simulink model "roachf_2048ch"  (Simulink 7.5)
settings: Solver=ode45  StartTime=0.0  StopTime=10.0  RelTol=1e-3
undefined symbols (not defined in the file or in its folder): Down, quant, ROACH, Up
libraries: xbsIndex_r4 x1405, xps_library x39, xbsReplacements_r4 x14, casper_library_misc x13, casper_library_delays x4, casper_library_sources x4, simulink x1
(part 1 of 14)
settings Model: Creator=zaki  LastModifiedBy=zaki
settings DebuggingCC: StrictBusMsg=Warning

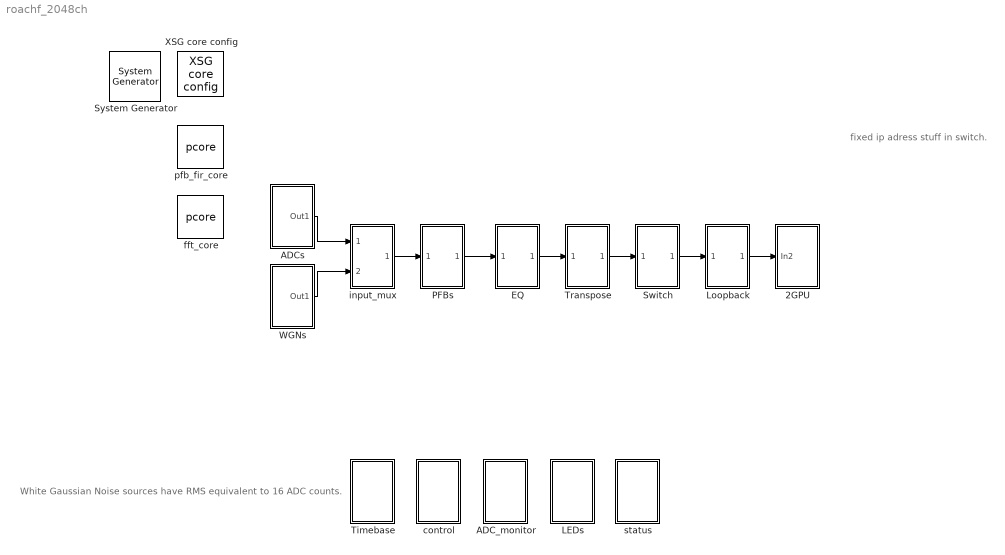
== system roachf_2048ch ==
  note: White Gaussian Noise
      | sources have RMS
      | equivalent to 16 ADC
      | counts.
  note: fixed ip adress stuff in switch.
  " System Generator" : xbsIndex_r4/ System Generator  Tag=genX  SystemSampleTime=-1  xilinxfamily=virtex5  part=xc5vsx95t  speed=-1  package=ff1136  synthesis_tool=XST  clock_wrapper=Clock Enables  directory=./roachf_2048ch/sysgen  proj_type=Project Navigator  Synth_file=XST Defaults  Impl_file=ISE Defaults  testbench=off  simulink_period=1  sysclk_period=5  dcm_input_clock_period=100  incr_netlist=off  trim_vbits=Everywhere in SubSystem  dbl_ovrd=According to Block Masks  core_generation=According to Block Masks  run_coregen=off  deprecated_control=off  eval_field=0  block_type=sysgen
      settings: block_version=10.1.3
  2GPU : Subsystem
  ADC_monitor : Subsystem
  ADCs : Subsystem
  EQ : Subsystem
  LEDs : Subsystem
  Loopback : Subsystem
  PFBs : Subsystem
  Switch : Subsystem
  Timebase : Subsystem
  Transpose : Subsystem
  WGNs : Subsystem
  XSG core config : xps_library/XSG core config  Tag=xps:xsg  SystemSampleTime=-1  hw_sys=ROACH:sx95t  ibob_linux=off  clk_src=adc0_clk  iBOB_clk_src=adc0_clk  BEE2_ctrl_clk_src=sys_clk  BEE2_usr_clk_src=sys_clk  ROACH_clk_src=adc0_clk  ROACH2_clk_src=adc0_clk  CORR_clk_src=sys_clk  gpio_clk_io_group=iBOB:sma  gpio_clk_bit_index=0  clk_rate=200  sample_period=1  synthesis_tool=XST  mpc_type=powerpc440_ext
  control : Subsystem
  fft_core : xps_library/pcore  Tag=xps:pcore  SystemSampleTime=-1  pcore_path=fft_core/fft_core.ngc
  input_mux : Subsystem
  pfb_fir_core : xps_library/pcore  Tag=xps:pcore  SystemSampleTime=-1  pcore_path=pfb_fir_core/pfb_fir_core.ngc
  status : Subsystem
  wires:
  ADCs/1(Out1) -> input_mux/1(In1)
  WGNs/1(Out1) -> input_mux/2(In2)
  input_mux/1(Out1) -> PFBs/1(In1)
  PFBs/1(Out1) -> EQ/1(In1)
  EQ/1(Out1) -> Transpose/1(In1)
  Transpose/1(Out1) -> Switch/1(In2)
  Switch/1(Out1) -> Loopback/1(In1)
  Loopback/1(Out1) -> 2GPU/1(In2)

== system roachf_2048ch/2GPU ==
  In2 : Inport
  10gbetxsnap : Subsystem  mask{nsamples=11}
      mask prompts: nsamples "Number of samples (2^?)"
  Constant1 : xbsIndex_r4/Constant  const=0  gui_display_data_type=Fixed-point  arith_type=Boolean  n_bits=16  bin_pt=14  preci_type=Single  exp_width=8  frac_width=24  explicit_period=on  period=1  equ=P=C  opselect=C  inp2=PCIN>>17  opr=+  inp1=P  carry=CIN  dbl_ovrd=off  block_type=constant
      settings: block_version=11.4
  Delay{,1..6} (7 alike) : xbsIndex_r4/Delay  rst=off  infoeditControl=Selection of Reset will increase slice count due to use of real FFs and instead of SRLs  en=off  latency=2  dbl_ovrd=off  reg_retiming=off  block_type=delay
  Inverter : xbsIndex_r4/Inverter  en=off  latency=0  dbl_ovrd=off  block_type=inv
      settings: block_version=11.4
  Inverter1 : xbsIndex_r4/Inverter  en=off  latency=0  dbl_ovrd=off  block_type=inv
  Logical : xbsIndex_r4/Logical  logical_function=AND  inputs=2  en=off  latency=0  precision=Full  arith_type=Unsigned  n_bits=16  bin_pt=0  align_bp=on  dbl_ovrd=off  block_type=logical
      settings: block_version=11.4
  Terminator : Terminator
  pack-it : Subsystem
  ten_GbE : xps_library/ten_GbE  Tag=xps:tengbe  SystemSampleTime=-1  port=ROACH:2  mac_lite=off  open_phy=off  show_param=off  pre_emph=3  swing=800  fab_en=off  fab_mac=0  fab_ip=0  fab_udp=0  fab_gate=0
  tag scope: gbe_gpu_led_rx=global, gbe_gpu_led_tx=global, gbe_gpu_led_up=global, gbe_gpu_rx_data=global, gbe_gpu_rx_eof=global, gbe_gpu_rx_ip=global, gbe_gpu_rx_port=global, gbe_gpu_rx_size=global, gbe_gpu_rx_valid=global, gbe_gpu_tx_ack=global
  wires:
  In2/1 -> Terminator/1
  [lb_mux_data] -> Delay/1
  [lb_mux_valid] -> Delay1/1
  [lb_mux_eof] -> Delay2/1
  [lb_mux_header] -> Delay3/1
  [lb_mux_flag] -> Delay4/1
  [lb_mux_err] -> Delay5/1
  [lb_mux_ip] -> Delay6/1
  [gpu_ip] -> ten_GbE/4
  [gpu_port] -> ten_GbE/5
  [data2gpu] -> ten_GbE/2
  pack-it/1(dataout) -> [data2gpu]
  pack-it/3(eof_out) -> [eof2gpu]
  pack-it/2(valid_out) -> [valid2gpu]
  [gbe_gpu_rst] -> ten_GbE/1
  Constant1/1 -> ten_GbE/8, ten_GbE/7
  [eof2gpu] -> ten_GbE/6
  ten_GbE/1 -> [gbe_gpu_led_up]
  ten_GbE/2 -> [gbe_gpu_led_rx]
  [gbe_gpu_disable] -> Inverter/1
  Inverter/1 -> Logical/1
  [valid2gpu] -> Logical/2
  Logical/1 -> 10gbetxsnap/2(valid_in), ten_GbE/3
  [data2gpu] -> 10gbetxsnap/1(data_in)
  [gpu_ip] -> 10gbetxsnap/3(ip_in)
  [eof2gpu] -> 10gbetxsnap/4(eof_in)
  [gbe_gpu_led_up] -> 10gbetxsnap/5(link_up)
  [gbe_gpu_led_tx] -> 10gbetxsnap/6(led_tx)
  [gbe_gpu_tx_ack] -> 10gbetxsnap/7(tx_ack)
  [gbe_gpu_tx_ack] -> Inverter1/1
  Delay/1 -> pack-it/1(data)
  Delay1/1 -> pack-it/2(valid)
  Delay2/1 -> pack-it/3(eof)
  Delay3/1 -> pack-it/4(header)
  Delay4/1 -> pack-it/5(flag)
  Delay5/1 -> pack-it/6(err)
  Delay6/1 -> pack-it/7(ip)
  ten_GbE/3 -> [gbe_gpu_led_tx]
  ten_GbE/4 -> [gbe_gpu_tx_ack]
  ten_GbE/5 -> [gbe_gpu_rx_data]
  ten_GbE/6 -> [gbe_gpu_rx_valid]
  ten_GbE/10 -> [gbe_gpu_rx_size]
  ten_GbE/7 -> [gbe_gpu_rx_ip]
  ten_GbE/8 -> [gbe_gpu_rx_port]
  ten_GbE/9 -> [gbe_gpu_rx_eof]
  Inverter1/1 -> 10gbetxsnap/8(tx_notack)

== system roachf_2048ch/ADC_monitor ==
  note: To provide a means for measuring the magnitude of the signals
      | coming in to each ADC channel, we have a "calc_adc_sum_sq"
      | block which uses a single multiplier, two accumulators, and two
      | regsiters to calculate the sum of 64K ADC samples and the sum
      | of squares of 64K ADC samples.  These can be used to calculate
      | the mean (aka DC offset) and standard deviation (aka RMS) of
      | the ADC inputs.
  note: adcN_levels are UFix_56_0.
      | The upper 16 bits are Fix_24_7 sum of samples.
      | The lower 32 bits are UFix_32_14 sum of squares.
  Counter : xbsIndex_r4/Counter  cnt_type=Free Running  cnt_to=Inf  operation=Up  start_count=0  cnt_by_val=1  arith_type=Unsigned  n_bits=16  bin_pt=0  load_pin=off  rst=off  en=off  explicit_period=off  period=1  dbl_ovrd=off  use_behavioral_HDL=off  implementation=Fabric  use_rpm=on  block_type=counter
      settings: xl_area=[0, 0, 0, 0, 0, 0, 0]
  Logical1 : xbsIndex_r4/Logical  logical_function=OR  inputs=8  en=off  latency=1  precision=Full  arith_type=Unsigned  n_bits=8  bin_pt=2  align_bp=on  dbl_ovrd=off  block_type=logical
      settings: xl_area=[0, 0, 0, 0, 0, 0, 0]
  Reinterpret{,1..7} (8 alike) : xbsIndex_r4/Reinterpret  force_arith_type=on  arith_type=Unsigned  force_bin_pt=on  bin_pt=0  block_type=reinterpret
      settings: infoedit="Changes signal type without altering the binary representation.   You can changed the signal between signed and unsigned, and relocate the binary point.<P><P>Hardware notes: In hardware this block costs nothing.<P><P>Example:  Suppose the input is 6 bits wide, signed, with 2 fractional bits, and the output is forced to unsigned with 0 fractional bits.  Then an input of -2.0 (1110.00 in binary 2's complement) becomes an output of 56 (111000 in binary)."  block_version=10.1.3
  Slice16 : xbsIndex_r4/Slice  nbits=1  boolean_output=on  mode=Upper Bit Location + Width  bit1=0  base1=MSB of Input  bit0=19  base0=LSB of Input  dbl_ovrd=off  block_type=slice
      settings: infoedit="Extracts a given range of bits from each input sample and presents it at the output.  The output type is ordinarily unsigned with binary point at zero, but can be Boolean when the slice is one bit wide.<P><P>Hardware notes: In hardware this block costs nothing."  block_version=10.1.3
  adc_clip_detect0 : Subsystem  mask{n_bits=8}
      mask prompts: n_bits "Number of ADC bits"
  adc_clip_detect1 : Subsystem  mask{n_bits=8}
      mask prompts: n_bits "Number of ADC bits"
  adc_clip_detect2 : Subsystem  mask{n_bits=8}
      mask prompts: n_bits "Number of ADC bits"
  adc_clip_detect3 : Subsystem  mask{n_bits=8}
      mask prompts: n_bits "Number of ADC bits"
  adc_clip_detect4 : Subsystem  mask{n_bits=8}
      mask prompts: n_bits "Number of ADC bits"
  adc_clip_detect5 : Subsystem  mask{n_bits=8}
      mask prompts: n_bits "Number of ADC bits"
  adc_clip_detect6 : Subsystem  mask{n_bits=8}
      mask prompts: n_bits "Number of ADC bits"
  adc_clip_detect7 : Subsystem  mask{n_bits=8}
      mask prompts: n_bits "Number of ADC bits"
  calc_adc_sum_sq0 : Subsystem
  calc_adc_sum_sq1 : Subsystem
  calc_adc_sum_sq2 : Subsystem
  calc_adc_sum_sq3 : Subsystem
  calc_adc_sum_sq4 : Subsystem
  calc_adc_sum_sq5 : Subsystem
  calc_adc_sum_sq6 : Subsystem
  calc_adc_sum_sq7 : Subsystem
  edge_detect : casper_library_misc/edge_detect  SystemSampleTime=-1  edge=Rising  polarity=Active High  x_in=[0 0.08 0.08 0.16 0.16 0.24 0.24 0.32 0.32 0.4]  y_in="[-1 -1  1  1  1  1  1  1  1  1]"  x_out=[0.6 0.68 0.68 0.76 0.76 0.84 0.84 0.92 0.92 1]  y_out="[-1 -1  1  1 -1 -1 -1 -1 -1 -1]"
  tag scope: adc_clip=global, in0_levels=global, in1_levels=global, in2_levels=global, in3_levels=global, in4_levels=global, in5_levels=global, in6_levels=global, in7_levels=global
  wires:
  [in0] -> calc_adc_sum_sq0/1(pol_in)
  calc_adc_sum_sq1/1(sum_sumsq) -> Reinterpret1/1
  calc_adc_sum_sq2/1(sum_sumsq) -> Reinterpret2/1
  calc_adc_sum_sq3/1(sum_sumsq) -> Reinterpret3/1
  edge_detect/1 -> calc_adc_sum_sq0/2(accum_rst), calc_adc_sum_sq1/2(accum_rst), calc_adc_sum_sq2/2(accum_rst), calc_adc_sum_sq3/2(accum_rst), calc_adc_sum_sq4/2(accum_rst), calc_adc_sum_sq5/2(accum_rst), calc_adc_sum_sq6/2(accum_rst), calc_adc_sum_sq7/2(accum_rst)
  [in1] -> calc_adc_sum_sq1/1(pol_in)
  [in2] -> calc_adc_sum_sq2/1(pol_in)
  [in3] -> calc_adc_sum_sq3/1(pol_in)
  Counter/1 -> Slice16/1
  Slice16/1 -> edge_detect/1
  calc_adc_sum_sq4/1(sum_sumsq) -> Reinterpret4/1
  [in4] -> calc_adc_sum_sq4/1(pol_in)
  calc_adc_sum_sq5/1(sum_sumsq) -> Reinterpret5/1
  calc_adc_sum_sq6/1(sum_sumsq) -> Reinterpret6/1
  calc_adc_sum_sq7/1(sum_sumsq) -> Reinterpret7/1
  [in5] -> calc_adc_sum_sq5/1(pol_in)
  [in6] -> calc_adc_sum_sq6/1(pol_in)
  [in7] -> calc_adc_sum_sq7/1(pol_in)
  Reinterpret/1 -> [in0_levels]
  Reinterpret1/1 -> [in1_levels]
  Reinterpret2/1 -> [in2_levels]
  Reinterpret3/1 -> [in3_levels]
  Reinterpret4/1 -> [in4_levels]
  Reinterpret5/1 -> [in5_levels]
  Reinterpret6/1 -> [in6_levels]
  Reinterpret7/1 -> [in7_levels]
  calc_adc_sum_sq0/1(sum_sumsq) -> Reinterpret/1
  [adc0] -> adc_clip_detect0/1(adc_in)
  [adc1] -> adc_clip_detect1/1(adc_in)
  [adc2] -> adc_clip_detect2/1(adc_in)
  [adc3] -> adc_clip_detect3/1(adc_in)
  [adc4] -> adc_clip_detect4/1(adc_in)
  [adc5] -> adc_clip_detect5/1(adc_in)
  [adc6] -> adc_clip_detect6/1(adc_in)
  [adc7] -> adc_clip_detect7/1(adc_in)
  adc_clip_detect0/1(clip) -> Logical1/1
  adc_clip_detect1/1(clip) -> Logical1/2
  adc_clip_detect2/1(clip) -> Logical1/3
  adc_clip_detect3/1(clip) -> Logical1/4
  adc_clip_detect4/1(clip) -> Logical1/5
  adc_clip_detect5/1(clip) -> Logical1/6
  adc_clip_detect6/1(clip) -> Logical1/7
  adc_clip_detect7/1(clip) -> Logical1/8
  Logical1/1 -> [adc_clip]

== system roachf_2048ch/ADCs ==
  Band-Limited White Noise : simulink/Sources/Band-Limited White Noise  SystemSampleTime=-1  Cov=[0.1]  Ts=0.1  seed=[23341]
  Constant : Constant  Value=0
  Constant1 : Constant
  Constant2 : Constant  Value=0
  Mux : Mux  Inputs=2
  Pulse Generator : DiscretePulseGenerator  Amplitude=1  Period=2^27  PulseWidth=1  PhaseDelay=0  SampleTime=1
  Terminator11 : Terminator
  Terminator12 : Terminator
  quadc0 : xps_library/quadc  Tag=xps:quadc  SystemSampleTime=-1  adc_brd=0  adc_clk_rate=200
  quadc1 : xps_library/quadc  Tag=xps:quadc  SystemSampleTime=-1  adc_brd=1  adc_clk_rate=200
  Out1 : Outport
  tag scope: adc0=global, adc1=global, adc2=global, adc3=global, adc4=global, adc5=global, adc6=global, adc7=global, sync_adc0=global, sync_adc1=global
  wires:
  quadc0/1 -> [adc0]
  quadc0/2 -> [adc1]
  quadc0/3 -> [adc2]
  quadc0/4 -> [adc3]
  quadc0/6 -> [sync_adc0]
  quadc1/1 -> [adc4]
  quadc1/2 -> [adc5]
  quadc1/3 -> [adc6]
  quadc1/4 -> [adc7]
  quadc1/6 -> [sync_adc1]
  Band-Limited White Noise/1 -> quadc1/4, quadc1/3, quadc1/2, quadc1/1, quadc0/4, quadc0/3, quadc0/2, quadc0/1
  Pulse Generator/1 -> quadc0/6, quadc1/6
  Constant1/1 -> quadc0/5, quadc1/5
  quadc0/5 -> Terminator11/1
  quadc1/5 -> Terminator12/1
  Mux/1 -> Out1/1
  Constant/1 -> Mux/1
  Constant2/1 -> Mux/2

== system roachf_2048ch/EQ ==
  note: Next, we reduce the bitwidth out of the FFT to 4 bits to save resources.
      | This must be done very carefully to avoid losing too much information.
      | Firstly, this conversion is done using "Round to Even" and saturation
      | logic to avoid introducing DC offsets, wrapping, and other ugly quantizaton
      | effects.  Secondly, the "equalizer" allows each frequency channel of the
      | FFT to be scaled by a different number.  This allows passbands which are
      | not flat to be flattened digitally to allow for optimal quantization to 4 bits.
      | These coefficients can also be updated dynamically for gain control.
      | Coefficients can be dynamically written into the "equalizer" by
      | specifying the channel ("coeff_addr") and the value of the
      | coefficient ("coeff"), and then using "coeff_en" to write the
      | new coefficient into the equalization table.
  note: eq_mon will monitor eq0, which consists of
      | in0 spectrum followed by in1 spectrum
  In1 : Inport
  Concat3 : xbsIndex_r4/Concat  num_inputs=4  dbl_ovrd=off  block_type=concat
      settings: block_version=10.1.3
  Logical5 : xbsIndex_r4/Logical  logical_function=OR  inputs=4  en=off  latency=0  precision=Full  arith_type=Unsigned  n_bits=8  bin_pt=2  align_bp=on  dbl_ovrd=off  block_type=logical
      settings: xl_area=[0, 0, 0, 0, 0, 0, 0]
  Terminator13 : Terminator
  Terminator14 : Terminator
  Terminator15 : Terminator
  eq0 : Subsystem
  eq1 : Subsystem
  eq2 : Subsystem
  eq3 : Subsystem
  Out1 : Outport
  tag scope: eq0=global, eq1=global, eq2=global, eq3=global, eq_clip0=global, eq_clip1=global, eq_clip2=global, eq_clip3=global, eq_clip=global, eq_mon=global, eq_out=global, sync_rnd=global
  wires:
  eq0/1(dout) -> [eq0], [eq_mon]
  eq0/2(sync_out) -> [sync_rnd]
  [fft0] -> eq0/1(in)
  [eq_data_0] -> eq0/3(coeff)
  [eq_en_0] -> eq0/4(coeff_we)
  eq0/3(clip) -> [eq_clip0]
  Logical5/1 -> [eq_clip]
  Concat3/1 -> [eq_out]
  [eq_clip0] -> Logical5/1
  [eq_clip1] -> Logical5/2
  [sync_fft0] -> eq0/2(sync)
  [eq_addr_0] -> eq0/5(coeff_addr)
  [fft1] -> eq1/1(in)
  [sync_fft0] -> eq1/2(sync)
  [eq_data_1] -> eq1/3(coeff)
  [eq_en_1] -> eq1/4(coeff_we)
  [eq_addr_1] -> eq1/5(coeff_addr)
  [fft2] -> eq2/1(in)
  [sync_fft0] -> eq2/2(sync)
  [eq_data_2] -> eq2/3(coeff)
  [eq_en_2] -> eq2/4(coeff_we)
  [eq_addr_2] -> eq2/5(coeff_addr)
  [fft3] -> eq3/1(in)
  [sync_fft0] -> eq3/2(sync)
  [eq_data_3] -> eq3/3(coeff)
  [eq_en_3] -> eq3/4(coeff_we)
  [eq_addr_3] -> eq3/5(coeff_addr)
  eq1/1(dout) -> [eq1]
  eq1/2(sync_out) -> Terminator13/1
  eq1/3(clip) -> [eq_clip1]
  eq2/1(dout) -> [eq2]
  eq2/2(sync_out) -> Terminator14/1
  eq2/3(clip) -> [eq_clip2]
  eq3/1(dout) -> [eq3]
  eq3/2(sync_out) -> Terminator15/1
  eq3/3(clip) -> [eq_clip3]
  [eq_clip2] -> Logical5/3
  [eq_clip3] -> Logical5/4
  [eq0] -> Concat3/1
  [eq1] -> Concat3/2
  [eq2] -> Concat3/3
  [eq3] -> Concat3/4
  In1/1 -> Out1/1

== system roachf_2048ch/LEDs ==
  Terminator{1..3,27} (4 alike) : Terminator
  led1_arm : xps_library/gpio  Tag=xps:gpio  SystemSampleTime=-1  io_group=ROACH:led  io_dir=out  arith_type=Boolean  bitwidth=1  bin_pt=0  bit_index=0  sample_period=1  use_single_ended=off  use_ddr=off  reg_iob=on  reg_clk_phase=0  termination=None
      link override convert: arith_type=Boolean  n_bits=1  bin_pt=0
  led2_sync : xps_library/gpio  Tag=xps:gpio  SystemSampleTime=-1  io_group=ROACH:led  io_dir=out  arith_type=Boolean  bitwidth=1  bin_pt=0  bit_index=1  sample_period=1  use_single_ended=off  use_ddr=off  reg_iob=on  reg_clk_phase=0  termination=None
      link override convert: arith_type=Boolean  n_bits=1  bin_pt=0
  led4_eq_clip : xps_library/gpio  Tag=xps:gpio  SystemSampleTime=-1  io_group=ROACH:led  io_dir=out  arith_type=Boolean  bitwidth=1  bin_pt=0  bit_index=2  sample_period=1  use_single_ended=off  use_ddr=off  reg_iob=on  reg_clk_phase=0  termination=None
      link override convert: arith_type=Boolean  n_bits=1  bin_pt=0
  led5_adc_clip : xps_library/gpio  Tag=xps:gpio  SystemSampleTime=-1  io_group=ROACH:led  io_dir=out  arith_type=Boolean  bitwidth=1  bin_pt=0  bit_index=3  sample_period=1  use_single_ended=off  use_ddr=off  reg_iob=on  reg_clk_phase=0  termination=None
      link override convert: arith_type=Boolean  n_bits=1  bin_pt=0
  pulse_ext2 : Subsystem  mask{pulse_len=2^23}
      mask prompts: pulse_len "Length of Pulse"
      mask init:
      | bits = ceil(log2(pulse_len+1));
  pulse_ext3 : Subsystem  mask{pulse_len=2^18}
      mask prompts: pulse_len "Length of Pulse"
      mask init:
      | bits = ceil(log2(pulse_len+1));
  pulse_ext4 : Subsystem  mask{pulse_len=2^18}
      mask prompts: pulse_len "Length of Pulse"
      mask init:
      | bits = ceil(log2(pulse_len+1));
  wires:
  pulse_ext2/1(out) -> led2_sync/1
  [sync_gen] -> pulse_ext2/1(in)
  [armed] -> led1_arm/1
  pulse_ext4/1(out) -> led4_eq_clip/1
  [eq_clip] -> pulse_ext4/1(in)
  led1_arm/1 -> Terminator27/1
  led4_eq_clip/1 -> Terminator2/1
  led2_sync/1 -> Terminator3/1
  [adc_clip] -> pulse_ext3/1(in)
  pulse_ext3/1(out) -> led5_adc_clip/1
  led5_adc_clip/1 -> Terminator1/1

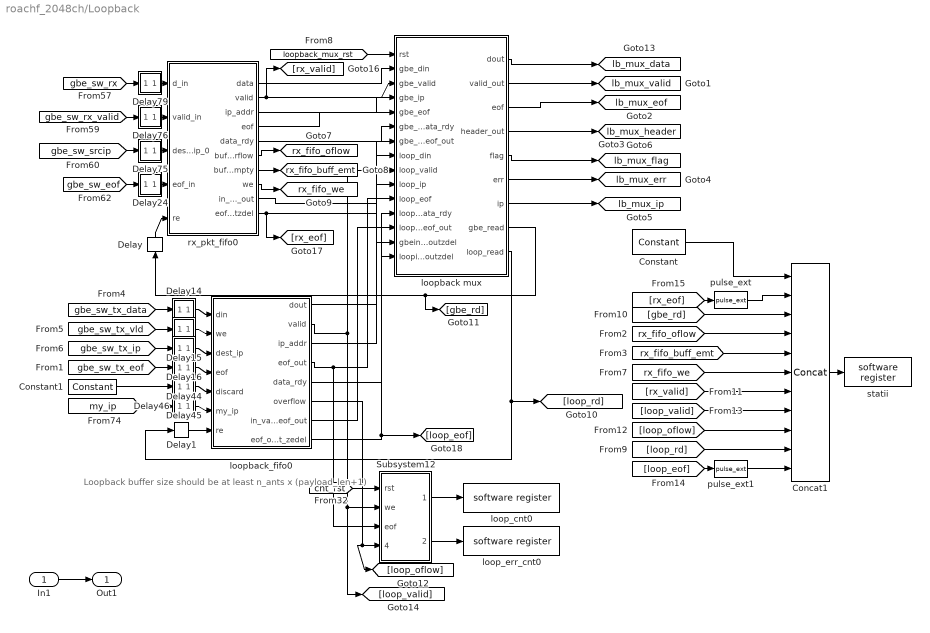
== system roachf_2048ch/Loopback ==
  note: Loopback buffer size should be at least
      | n_ants x (payload_len+1)
  In1 : Inport
  Concat1 : xbsIndex_r4/Concat  num_inputs=11  dbl_ovrd=off  block_type=concat
  Constant : xbsIndex_r4/Constant  const=0  gui_display_data_type=Fixed-point  arith_type=Unsigned  n_bits=22  bin_pt=0  preci_type=Single  exp_width=8  frac_width=24  explicit_period=on  period=1  equ=P=C  opselect=C  inp2=PCIN>>17  opr=+  inp1=P  carry=CIN  dbl_ovrd=off  block_type=constant
      settings: block_version=11.4
  Constant1 : xbsIndex_r4/Constant  const=0  gui_display_data_type=Boolean  arith_type=Boolean  n_bits=1  bin_pt=0  preci_type=Single  exp_width=8  frac_width=24  explicit_period=on  period=1  equ=P=C  opselect=C  inp2=PCIN>>17  opr=+  inp1=P  carry=CIN  dbl_ovrd=off  block_type=constant
      settings: block_version=11.4
  Delay : xbsIndex_r4/Delay  rst=off  infoeditControl=Selection of Reset will increase slice count due to use of real FFs and instead of SRLs  en=off  latency=1  dbl_ovrd=off  reg_retiming=off  block_type=delay
  Delay1 : xbsIndex_r4/Delay  rst=off  infoeditControl=Selection of Reset will increase slice count due to use of real FFs and instead of SRLs  en=off  latency=1  dbl_ovrd=off  reg_retiming=off  block_type=delay
  Delay14 : Subsystem  AncestorBlock=casper_library/Delays/pipeline  mask(pipeline){latency=1}
      mask help:
      | An explicitly laid-out delay line to avoid mapping to SRL16s
      | for use in pipelining to help achieve timing closure.
      mask init:
      | pipeline_init(gcb, 'latency', latency);
      mask Display:
      | port_label('input', 1, 'd');
      | port_label('output', 1, 'q');
      | disp(['Z^-', num2str(latency)]);
  Delay15 : Subsystem  AncestorBlock=casper_library/Delays/pipeline  mask(pipeline){latency=1}
      mask help:
      | An explicitly laid-out delay line to avoid mapping to SRL16s
      | for use in pipelining to help achieve timing closure.
      mask init:
      | pipeline_init(gcb, 'latency', latency);
      mask Display:
      | port_label('input', 1, 'd');
      | port_label('output', 1, 'q');
      | disp(['Z^-', num2str(latency)]);
  Delay16 : Subsystem  AncestorBlock=casper_library/Delays/pipeline  mask(pipeline){latency=1}
      mask help:
      | An explicitly laid-out delay line to avoid mapping to SRL16s
      | for use in pipelining to help achieve timing closure.
      mask init:
      | pipeline_init(gcb, 'latency', latency);
      mask Display:
      | port_label('input', 1, 'd');
      | port_label('output', 1, 'q');
      | disp(['Z^-', num2str(latency)]);
  Delay24 : Subsystem  AncestorBlock=casper_library/Delays/pipeline  mask(pipeline){latency=1}
      mask help:
      | An explicitly laid-out delay line to avoid mapping to SRL16s
      | for use in pipelining to help achieve timing closure.
      mask init:
      | pipeline_init(gcb, 'latency', latency);
      mask Display:
      | port_label('input', 1, 'd');
      | port_label('output', 1, 'q');
      | disp(['Z^-', num2str(latency)]);
  Delay44 : Subsystem  AncestorBlock=casper_library/Delays/pipeline  mask(pipeline){latency=1}
      mask help:
      | An explicitly laid-out delay line to avoid mapping to SRL16s
      | for use in pipelining to help achieve timing closure.
      mask init:
      | pipeline_init(gcb, 'latency', latency);
      mask Display:
      | port_label('input', 1, 'd');
      | port_label('output', 1, 'q');
      | disp(['Z^-', num2str(latency)]);
  Delay45 : Subsystem  AncestorBlock=casper_library/Delays/pipeline  mask(pipeline){latency=1}
      mask help:
      | An explicitly laid-out delay line to avoid mapping to SRL16s
      | for use in pipelining to help achieve timing closure.
      mask init:
      | pipeline_init(gcb, 'latency', latency);
      mask Display:
      | port_label('input', 1, 'd');
      | port_label('output', 1, 'q');
      | disp(['Z^-', num2str(latency)]);
  Delay46 : Subsystem  AncestorBlock=casper_library/Delays/pipeline  mask(pipeline){latency=1}
      mask help:
      | An explicitly laid-out delay line to avoid mapping to SRL16s
      | for use in pipelining to help achieve timing closure.
      mask init:
      | pipeline_init(gcb, 'latency', latency);
      mask Display:
      | port_label('input', 1, 'd');
      | port_label('output', 1, 'q');
      | disp(['Z^-', num2str(latency)]);
  Delay75 : Subsystem  AncestorBlock=casper_library/Delays/pipeline  mask(pipeline){latency=1}
      mask help:
      | An explicitly laid-out delay line to avoid mapping to SRL16s
      | for use in pipelining to help achieve timing closure.
      mask init:
      | pipeline_init(gcb, 'latency', latency);
      mask Display:
      | port_label('input', 1, 'd');
      | port_label('output', 1, 'q');
      | disp(['Z^-', num2str(latency)]);
  Delay76 : Subsystem  AncestorBlock=casper_library/Delays/pipeline  mask(pipeline){latency=1}
      mask help:
      | An explicitly laid-out delay line to avoid mapping to SRL16s
      | for use in pipelining to help achieve timing closure.
      mask init:
      | pipeline_init(gcb, 'latency', latency);
      mask Display:
      | port_label('input', 1, 'd');
      | port_label('output', 1, 'q');
      | disp(['Z^-', num2str(latency)]);
  Delay79 : Subsystem  AncestorBlock=casper_library/Delays/pipeline  mask(pipeline){latency=1}
      mask help:
      | An explicitly laid-out delay line to avoid mapping to SRL16s
      | for use in pipelining to help achieve timing closure.
      mask init:
      | pipeline_init(gcb, 'latency', latency);
      mask Display:
      | port_label('input', 1, 'd');
      | port_label('output', 1, 'q');
      | disp(['Z^-', num2str(latency)]);
  Subsystem12 : Subsystem
  loop_cnt0 : xps_library/software register  Tag=xps:sw_reg  SystemSampleTime=-1  io_dir=To Processor  arith_type=Unsigned  bitwidth=32  bin_pt=0  sample_period=1  gw_name=roachf_2048ch_Loopback_loop_cnt0_user_data_in
      link override convert: arith_type=Unsigned  n_bits=32  bin_pt=0
  loop_err_cnt0 : xps_library/software register  Tag=xps:sw_reg  SystemSampleTime=-1  io_dir=To Processor  arith_type=Unsigned  bitwidth=32  bin_pt=0  sample_period=1  gw_name=roachf_2048ch_Loopback_loop_err_cnt0_user_data_in
      link override convert: arith_type=Unsigned  n_bits=32  bin_pt=0
  loopback mux : Subsystem
  loopback_fifo0 : Subsystem
  pulse_ext : casper_library_misc/pulse_ext  SystemSampleTime=-1  pulse_len=512
  pulse_ext1 : casper_library_misc/pulse_ext  SystemSampleTime=-1  pulse_len=512
  rx_pkt_fifo0 : Subsystem
      settings: AttributesFormatString=|
      | Max 1024 data words.
      | Max 32 pkts.
  statii : xps_library/software register  Tag=xps:sw_reg  SystemSampleTime=-1  io_dir=To Processor  arith_type=Unsigned  bitwidth=32  bin_pt=0  sample_period=1  gw_name=roachf_2048ch_Loopback_statii_user_data_in
      link override convert: arith_type=Unsigned  n_bits=32  bin_pt=0
  Out1 : Outport
  tag scope: lb_mux_data=global, lb_mux_eof=global, lb_mux_err=global, lb_mux_flag=global, lb_mux_header=global, lb_mux_ip=global, lb_mux_valid=global, rx_fifo_buff_emt=global, rx_fifo_oflow=global, rx_fifo_we=global
  wires:
  loopback_fifo0/2(valid) -> loopback mux/9(loop_valid), Subsystem12/2(we), [loop_valid]
  rx_pkt_fifo0/1(data) -> loopback mux/2(gbe_din)
  rx_pkt_fifo0/2(valid) -> loopback mux/3(gbe_valid), [rx_valid]
  [cnt_rst] -> Subsystem12/1(rst)
  Subsystem12/2(err_cnt) -> loop_err_cnt0/1
  Subsystem12/1(rx_cnt) -> loop_cnt0/1
  [loopback_mux_rst] -> loopback mux/1(rst)
  [gbe_sw_srcip] -> Delay75/1(d)
  [gbe_sw_rx_valid] -> Delay76/1(d)
  [gbe_sw_rx] -> Delay79/1(d)
  [gbe_sw_eof] -> Delay24/1(d)
  Delay79/1(q) -> rx_pkt_fifo0/1(d_in)
  Delay76/1(q) -> rx_pkt_fifo0/2(valid_in)
  Delay75/1(q) -> rx_pkt_fifo0/3(dest_ip_0)
  Delay24/1(q) -> rx_pkt_fifo0/4(eof_in)
  [my_ip] -> Delay46/1(d)
  [gbe_sw_tx_data] -> Delay14/1(d)
  [gbe_sw_tx_vld] -> Delay15/1(d)
  [gbe_sw_tx_ip] -> Delay16/1(d)
  [gbe_sw_tx_eof] -> Delay44/1(d)
  Constant1/1 -> Delay45/1(d)
  Delay14/1(q) -> loopback_fifo0/1(din)
  Delay15/1(q) -> loopback_fifo0/2(we)
  Delay16/1(q) -> loopback_fifo0/3(dest_ip)
  Delay44/1(q) -> loopback_fifo0/4(eof)
  Delay45/1(q) -> loopback_fifo0/5(discard)
  Delay46/1(q) -> loopback_fifo0/6(my_ip)
  In1/1 -> Out1/1
  loopback mux/1(dout) -> [lb_mux_data]
  loopback mux/2(valid_out) -> [lb_mux_valid]
  loopback mux/5(flag) -> [lb_mux_flag]
  loopback mux/6(err) -> [lb_mux_err]
  Concat1/1 -> statii/1
  loopback mux/3(eof) -> [lb_mux_eof]
  loopback mux/4(header_out) -> [lb_mux_header]
  loopback mux/7(ip) -> [lb_mux_ip]
  loopback mux/9(loop_read) -> Delay1/1, [loop_rd]
  loopback_fifo0/4(eof_out) -> Subsystem12/3(eof), loopback mux/11(loop_eof)
  loopback_fifo0/6(overflow) -> Subsystem12/4(overflow), [loop_oflow]
  rx_pkt_fifo0/6(buffer_overflow) -> [rx_fifo_oflow]
  rx_pkt_fifo0/7(buffer_empty) -> [rx_fifo_buff_emt]
  rx_pkt_fifo0/8(we) -> [rx_fifo_we]
  loopback mux/8(gbe_read) -> Delay/1, [gbe_rd]
  rx_pkt_fifo0/4(eof) -> loopback mux/5(gbe_eof)
  rx_pkt_fifo0/3(ip_addr) -> loopback mux/4(gbe_ip)
  rx_pkt_fifo0/5(data_rdy) -> loopback mux/6(gbe_data_rdy)
  rx_pkt_fifo0/9(in_valid_eof_out) -> loopback mux/7(gbe_in_valid_eof_out)
  loopback_fifo0/1(dout) -> loopback mux/8(loop_din)
  loopback_fifo0/3(ip_addr) -> loopback mux/10(loop_ip)
  loopback_fifo0/5(data_rdy) -> loopback mux/12(loop_data_rdy)
  loopback_fifo0/7(in_valid_eof_out) -> loopback mux/13(loop_in_valid_eof_out)
  rx_pkt_fifo0/10(eofoutzdel) -> loopback mux/14(gbeineofoutzdel), [rx_eof]
  loopback_fifo0/8(eof_out_zedel) -> loopback mux/15(loopineofoutzdel), [loop_eof]
  Delay/1 -> rx_pkt_fifo0/5(re)
  Delay1/1 -> loopback_fifo0/7(re)
  [rx_eof] -> pulse_ext/1
  [loop_eof] -> pulse_ext1/1
  pulse_ext1/1 -> Concat1/11
  [loop_rd] -> Concat1/10
  [loop_oflow] -> Concat1/9
  [loop_valid] -> Concat1/8
  [rx_valid] -> Concat1/7
  [rx_fifo_we] -> Concat1/6
  [rx_fifo_buff_emt] -> Concat1/5
  [rx_fifo_oflow] -> Concat1/4
  [gbe_rd] -> Concat1/3
  pulse_ext/1 -> Concat1/2
  Constant/1 -> Concat1/1

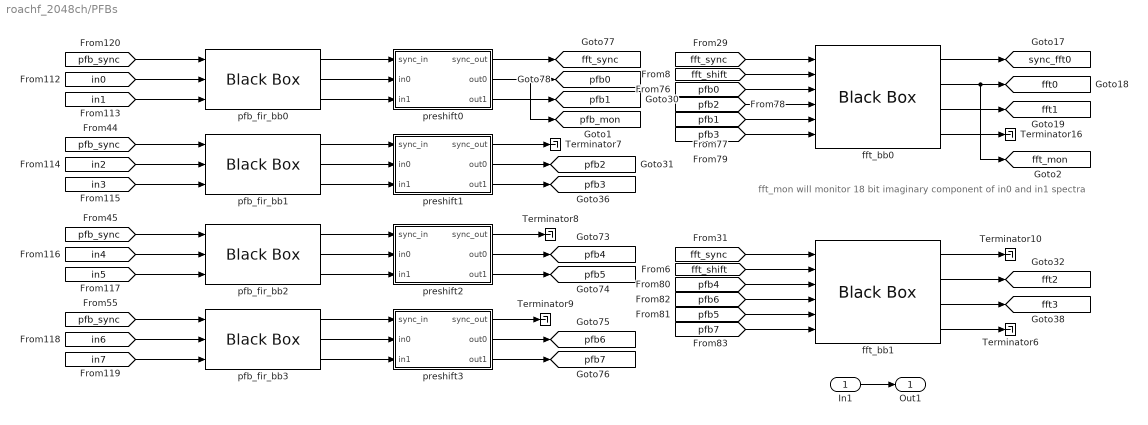
== system roachf_2048ch/PFBs ==
  note: fft_mon will monitor 18 bit imaginary component of in0 and in1 spectra
  In1 : Inport
  Terminator{6..10,16} (6 alike) : Terminator
  fft_bb0 : xbsIndex_r4/Black Box  init_code=fft_core_config  sim_method=Inactive  verbose=off  block_type=blackbox2
      settings: infoedit="Incorporates black box HDL and simulation model into a System Generator design.<P><P>You must supply a Black Box with certain information about the HDL component you would like to bring into System Generator. This information is provided through a Matlab function.<P><P>When \"Simulation mode\" is set to \"Inactive\", you will typically want to provide a separate simulation model by using a Simulation Multiplexer.<P>When \"Simulation mode\" is set to \"External co-simulator\", you must include a ModelSim block in the design."  block_version=10.1.3
  fft_bb1 : xbsIndex_r4/Black Box  init_code=fft_core_config  sim_method=Inactive  verbose=off  block_type=blackbox2
      settings: infoedit="Incorporates black box HDL and simulation model into a System Generator design.<P><P>You must supply a Black Box with certain information about the HDL component you would like to bring into System Generator. This information is provided through a Matlab function.<P><P>When \"Simulation mode\" is set to \"Inactive\", you will typically want to provide a separate simulation model by using a Simulation Multiplexer.<P>When \"Simulation mode\" is set to \"External co-simulator\", you must include a ModelSim block in the design."  block_version=10.1.3
  pfb_fir_bb{0..3} (4 alike) : xbsIndex_r4/Black Box  init_code=pfb_fir_core_config  sim_method=Inactive  verbose=off  block_type=blackbox2
      settings: infoedit="Incorporates black box HDL and simulation model into a System Generator design.<P><P>You must supply a Black Box with certain information about the HDL component you would like to bring into System Generator. This information is provided through a Matlab function.<P><P>When \"Simulation mode\" is set to \"Inactive\", you will typically want to provide a separate simulation model by using a Simulation Multiplexer.<P>When \"Simulation mode\" is set to \"External co-simulator\", you must include a ModelSim block in the design."  block_version=10.1.3
  preshift0 : Subsystem
  preshift1 : Subsystem
  preshift2 : Subsystem
  preshift3 : Subsystem
  Out1 : Outport
  tag scope: fft0=global, fft1=global, fft2=global, fft3=global, fft_mon=global, fft_sync=global, pfb0=global, pfb1=global, pfb2=global, pfb3=global, pfb4=global, pfb5=global, pfb6=global, pfb7=global, pfb_mon=global, sync_fft0=global
  wires:
  [in0] -> pfb_fir_bb0/2
  [in1] -> pfb_fir_bb0/3
  [in2] -> pfb_fir_bb1/2
  [in3] -> pfb_fir_bb1/3
  [in4] -> pfb_fir_bb2/2
  [in5] -> pfb_fir_bb2/3
  [in6] -> pfb_fir_bb3/2
  [in7] -> pfb_fir_bb3/3
  pfb_fir_bb1/2 -> preshift1/2(in0)
  pfb_fir_bb1/3 -> preshift1/3(in1)
  pfb_fir_bb2/2 -> preshift2/2(in0)
  pfb_fir_bb2/3 -> preshift2/3(in1)
  pfb_fir_bb3/2 -> preshift3/2(in0)
  pfb_fir_bb3/3 -> preshift3/3(in1)
  [fft_sync] -> fft_bb1/1
  [fft_shift] -> fft_bb1/2
  fft_bb1/3 -> [fft3]
  fft_bb1/4 -> Terminator6/1
  fft_bb1/2 -> [fft2]
  fft_bb0/2 -> [fft0], [fft_mon]
  fft_bb0/3 -> [fft1]
  fft_bb0/4 -> Terminator16/1
  fft_bb0/1 -> [sync_fft0]
  fft_bb1/1 -> Terminator10/1
  [pfb0] -> fft_bb0/3
  [pfb2] -> fft_bb0/4
  [pfb1] -> fft_bb0/5
  [pfb3] -> fft_bb0/6
  [fft_sync] -> fft_bb0/1
  [fft_shift] -> fft_bb0/2
  [pfb4] -> fft_bb1/3
  [pfb6] -> fft_bb1/4
  [pfb5] -> fft_bb1/5
  [pfb7] -> fft_bb1/6
  [pfb_sync] -> pfb_fir_bb0/1
  [pfb_sync] -> pfb_fir_bb1/1
  [pfb_sync] -> pfb_fir_bb2/1
  [pfb_sync] -> pfb_fir_bb3/1
  pfb_fir_bb1/1 -> preshift1/1(sync_in)
  pfb_fir_bb2/1 -> preshift2/1(sync_in)
  pfb_fir_bb3/1 -> preshift3/1(sync_in)
  In1/1 -> Out1/1
  pfb_fir_bb0/1 -> preshift0/1(sync_in)
  pfb_fir_bb0/2 -> preshift0/2(in0)
  pfb_fir_bb0/3 -> preshift0/3(in1)
  preshift0/1(sync_out) -> [fft_sync]
  preshift0/2(out0) -> [pfb0], [pfb_mon]
  preshift0/3(out1) -> [pfb1]
  preshift1/1(sync_out) -> Terminator7/1
  preshift2/1(sync_out) -> Terminator8/1
  preshift3/1(sync_out) -> Terminator9/1
  preshift1/2(out0) -> [pfb2]
  preshift1/3(out1) -> [pfb3]
  preshift2/2(out0) -> [pfb4]
  preshift2/3(out1) -> [pfb5]
  preshift3/2(out0) -> [pfb6]
  preshift3/3(out1) -> [pfb7]

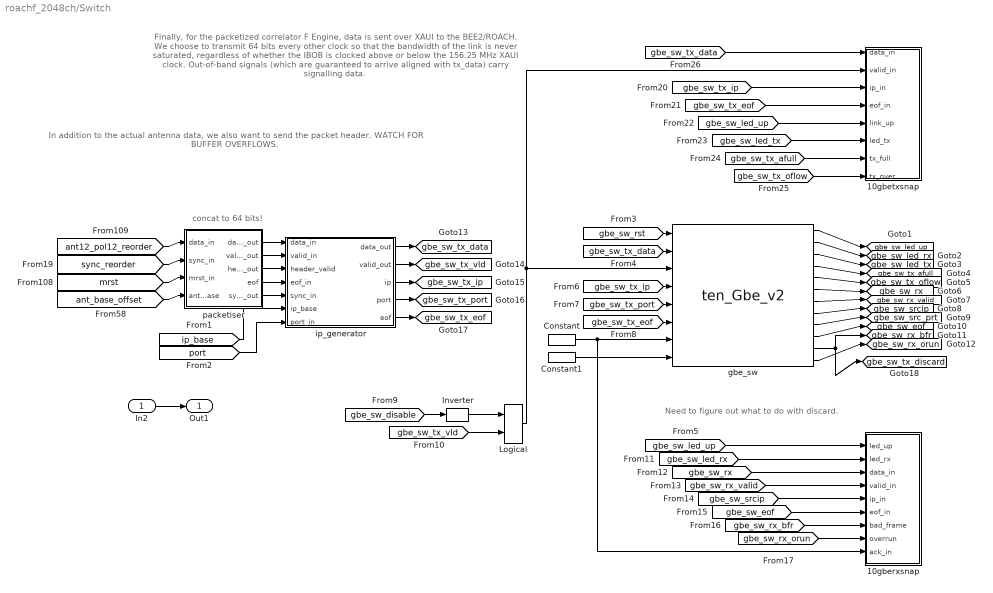
== system roachf_2048ch/Switch ==
  note: Finally, for the packetized correlator F Engine, data is sent over
      | XAUI to the BEE2/ROACH.  We choose to transmit 64 bits every other clock
      | so that the bandwidth of the link is never saturated, regardless of whether
      | the IBOB is clocked above or below the 156.25 MHz XAUI clock.
      | Out-of-band signals (which are guaranteed to arrive aligned with
      | tx_data) carry signalling data.
  note: In addition to the actual antenna data,
      | we also want to send the packet header.
      | WATCH FOR BUFFER OVERFLOWS.
  note: concat to 64 bits!
  note: Need to figure out what to do with discard.
  In2 : Inport
  10gberxsnap : Subsystem  mask{nsamples=10}
      mask prompts: nsamples "Number of samples (2^?)"
  10gbetxsnap : Subsystem  mask{nsamples=10}
      mask prompts: nsamples "Number of samples (2^?)"
  Constant : xbsIndex_r4/Constant  const=1  gui_display_data_type=Fixed-point  arith_type=Boolean  n_bits=16  bin_pt=14  preci_type=Single  exp_width=8  frac_width=24  explicit_period=on  period=1  equ=P=C  opselect=C  inp2=PCIN>>17  opr=+  inp1=P  carry=CIN  dbl_ovrd=off  block_type=constant
      settings: block_version=11.4
  Constant1 : xbsIndex_r4/Constant  const=0  gui_display_data_type=Fixed-point  arith_type=Boolean  n_bits=16  bin_pt=14  preci_type=Single  exp_width=8  frac_width=24  explicit_period=on  period=1  equ=P=C  opselect=C  inp2=PCIN>>17  opr=+  inp1=P  carry=CIN  dbl_ovrd=off  block_type=constant
      settings: block_version=11.4
  Inverter : xbsIndex_r4/Inverter  en=off  latency=0  dbl_ovrd=off  block_type=inv
      settings: block_version=11.4
  Logical : xbsIndex_r4/Logical  logical_function=AND  inputs=2  en=off  latency=0  precision=Full  arith_type=Unsigned  n_bits=16  bin_pt=0  align_bp=on  dbl_ovrd=off  block_type=logical
      settings: block_version=11.4
  gbe_sw : xps_library/ten_Gbe_v2  Tag=xps:tengbe_v2  SystemSampleTime=-1  port=3  rx_dist_ram=off  large_frames=on  show_param=off  pre_emph=3  swing=800  fab_en=off  fab_mac=hex2dec('123456780000')  fab_ip=192*(2^24) + 168*(2^16) + 5*(2^8) + 20*(2^0)  fab_udp=10000  fab_gate=1  cpu_rx_en=on  cpu_tx_en=on
  ip_generator : Subsystem
  packetiser : Subsystem  mask{nwrd_bits=10, ant_bits=2, nSpec=2, nXeng=3, nChan=11}
      mask prompts: nwrd_bits "Payload length: (in 64bit words) (2^n)"; ant_bits "Number of antennas on this link (2^n)"; nSpec "Number of spectra(time samples) to acc. (2^?)"; nXeng "Number of Xengines total (2^?)"; nChan "Number of Channels in a spectra(2^?)"
      mask help: Package 32 bit data into 64 bits and identify data as coming from antenna 0 or 1
  Out1 : Outport
  tag scope: gbe_sw_eof=global, gbe_sw_led_rx=global, gbe_sw_led_tx=global, gbe_sw_led_up=global, gbe_sw_rx=global, gbe_sw_rx_bfr=global, gbe_sw_rx_orun=global, gbe_sw_rx_valid=global, gbe_sw_src_prt=global, gbe_sw_srcip=global, gbe_sw_tx_afull=global, gbe_sw_tx_data=global, gbe_sw_tx_discard=global, gbe_sw_tx_eof=global, gbe_sw_tx_ip=global, gbe_sw_tx_oflow=global, gbe_sw_tx_port=global, gbe_sw_tx_vld=global
  wires:
  [sync_reorder] -> packetiser/2(sync_in)
  [mrst] -> packetiser/3(mrst_in)
  [ant12_pol12_reorder] -> packetiser/1(data_in)
  [ant_base_offset] -> packetiser/4(ant_base)
  packetiser/5(sync_out) -> ip_generator/5(sync_in)
  packetiser/4(eof) -> ip_generator/4(eof_in)
  packetiser/3(header_out) -> ip_generator/3(header_valid)
  packetiser/2(valid_out) -> ip_generator/2(valid_in)
  packetiser/1(data_out) -> ip_generator/1(data_in)
  In2/1 -> Out1/1
  [ip_base] -> ip_generator/6(ip_base)
  [port] -> ip_generator/7(port_in)
  [gbe_sw_rst] -> gbe_sw/1
  gbe_sw/1 -> [gbe_sw_led_up]
  gbe_sw/2 -> [gbe_sw_led_rx]
  gbe_sw/3 -> [gbe_sw_led_tx]
  gbe_sw/4 -> [gbe_sw_tx_afull]
  gbe_sw/5 -> [gbe_sw_tx_oflow]
  gbe_sw/6 -> [gbe_sw_rx]
  gbe_sw/7 -> [gbe_sw_rx_valid]
  gbe_sw/8 -> [gbe_sw_srcip]
  gbe_sw/9 -> [gbe_sw_src_prt]
  gbe_sw/10 -> [gbe_sw_eof]
  gbe_sw/11 -> [gbe_sw_rx_bfr], [gbe_sw_tx_discard]
  gbe_sw/12 -> [gbe_sw_rx_orun]
  ip_generator/1(data_out) -> [gbe_sw_tx_data]
  ip_generator/2(valid_out) -> [gbe_sw_tx_vld]
  ip_generator/3(ip) -> [gbe_sw_tx_ip]
  ip_generator/4(port) -> [gbe_sw_tx_port]
  ip_generator/5(eof) -> [gbe_sw_tx_eof]
  Constant/1 -> gbe_sw/7, 10gberxsnap/9(ack_in)
  Constant1/1 -> gbe_sw/8
  [gbe_sw_tx_data] -> gbe_sw/2
  Logical/1 -> gbe_sw/3, 10gbetxsnap/2(valid_in)
  [gbe_sw_tx_ip] -> gbe_sw/4
  [gbe_sw_tx_port] -> gbe_sw/5
  [gbe_sw_tx_eof] -> gbe_sw/6
  [gbe_sw_disable] -> Inverter/1
  Inverter/1 -> Logical/1
  [gbe_sw_tx_vld] -> Logical/2
  [gbe_sw_led_up] -> 10gberxsnap/1(led_up)
  [gbe_sw_led_rx] -> 10gberxsnap/2(led_rx)
  [gbe_sw_rx] -> 10gberxsnap/3(data_in)
  [gbe_sw_rx_valid] -> 10gberxsnap/4(valid_in)
  [gbe_sw_srcip] -> 10gberxsnap/5(ip_in)
  [gbe_sw_eof] -> 10gberxsnap/6(eof_in)
  [gbe_sw_rx_bfr] -> 10gberxsnap/7(bad_frame)
  [gbe_sw_rx_orun] -> 10gberxsnap/8(overrun)
  [gbe_sw_led_tx] -> 10gbetxsnap/6(led_tx)
  [gbe_sw_tx_afull] -> 10gbetxsnap/7(tx_full)
  [gbe_sw_tx_oflow] -> 10gbetxsnap/8(tx_over)
  [gbe_sw_led_up] -> 10gbetxsnap/5(link_up)
  [gbe_sw_tx_eof] -> 10gbetxsnap/4(eof_in)
  [gbe_sw_tx_data] -> 10gbetxsnap/1(data_in)
  [gbe_sw_tx_ip] -> 10gbetxsnap/3(ip_in)

== system roachf_2048ch/Timebase ==
  note: This circuit implements a scheme for synchronizing
      | multiple IBOBs to within a 200 MHz clock.  "arm_rst"
      | comes from the "ctrl" register, and indicates that the
      | next "sync_rst" should reset the sync pulse generated
      | in "sync_gen".  "sync_rst" may be generated from
      | the "ctrl" register, but more often, a 1PPS signal is
      | supplied to the "sync" input of an ADC for this
      | purpose.  Once a reset occurs, "sync_gen" generates
      | a single pulse every 2^27 clocks.  LEDs provide visual
      | confirmation that an arm and reset occur, and "mrst"
      | is passed over XAUI for the purpose of informing
      | downstream logic in a packetized correlator that
      | a "master reset" has occurred.
  Logical7 : xbsIndex_r4/Logical  logical_function=OR  inputs=3  en=off  latency=1  precision=Full  arith_type=Unsigned  n_bits=8  bin_pt=2  align_bp=on  dbl_ovrd=off  block_type=logical
      settings: xl_area=[0, 0, 0, 0, 0, 0, 0]
  sync_gen : Subsystem
  tag scope: armed=global, mrst=global, sync_gen=global
  wires:
  sync_gen/1(sync) -> [sync_gen]
  sync_gen/2(mrst) -> [mrst]
  [arm_rst] -> sync_gen/2(arm)
  [sync_rst] -> Logical7/2
  sync_gen/3(armed) -> [armed]
  Logical7/1 -> sync_gen/1(rst)
  [sync_adc0] -> Logical7/1
  [sync_adc1] -> Logical7/3

== system roachf_2048ch/Transpose ==
  note: A matrix transpose is performed in SRAM so that 128 samples of frequency
      | channel 0 are output, followed by 128 samples of channel 1, and so forth.
      | These blocks of samples for a single channel are turned into 10 GbE packets
      | on the X engine, and are then routed through a swittch.  "one_ant_a_time"
      | outputs 128 samples for channel 0 (both polarizations) of one antenna,
      | and then 128 samples for channel 0 of the other antenna, followed by
      | channel 1 of the first antenna, and so on.  This allows the X engine design to
      | pass data directly from the XAUI into a packet containing 128 time samples
      | for 1 frequency from 1 antenna.
  note: Currently "dbuf_ct_sram" double-buffers data (meaning it writes data
      | into one buffer, while reading data out in the desired order from another
      | buffer.  Look into QDR or bigger BRAMS to increas number of channels.
  note: A matrix transpose and reorder is performed in Shared BRAMS.
      | Currently, 8 time samples of frequency%16 are output. for #channels = 2048
      | 128 channels (the channels to be sent to one xengine, in order 0,16,32,...for xengine0.
      | ch#1,17,33... for xeng1. etc..)
      | That is ch(mod16) = i gets sent to xengine i (wherever it maybe located).
      | One ant at a time fixes interleaving of all 4 antennas on one roach. That is it takes
      | output of transpose and sends all antennas for a single channel,all time samples. then starts
      | new channel. etc.... (see old comment below).
  In1 : Inport
  Delay1 : Subsystem  AncestorBlock=casper_library/Delays/pipeline  mask(pipeline){latency=1}
      mask help:
      | An explicitly laid-out delay line to avoid mapping to SRL16s
      | for use in pipelining to help achieve timing closure.
      mask init:
      | pipeline_init(gcb, 'latency', latency);
      mask Display:
      | port_label('input', 1, 'd');
      | port_label('output', 1, 'q');
      | disp(['Z^-', num2str(latency)]);
  Delay2 : Subsystem  AncestorBlock=casper_library/Delays/pipeline  mask(pipeline){latency=1}
      mask help:
      | An explicitly laid-out delay line to avoid mapping to SRL16s
      | for use in pipelining to help achieve timing closure.
      mask init:
      | pipeline_init(gcb, 'latency', latency);
      mask Display:
      | port_label('input', 1, 'd');
      | port_label('output', 1, 'q');
      | disp(['Z^-', num2str(latency)]);
  Delay3 : Subsystem  AncestorBlock=casper_library/Delays/pipeline  mask(pipeline){latency=1}
      mask help:
      | An explicitly laid-out delay line to avoid mapping to SRL16s
      | for use in pipelining to help achieve timing closure.
      mask init:
      | pipeline_init(gcb, 'latency', latency);
      mask Display:
      | port_label('input', 1, 'd');
      | port_label('output', 1, 'q');
      | disp(['Z^-', num2str(latency)]);
  Delay79 : Subsystem  AncestorBlock=casper_library/Delays/pipeline  mask(pipeline){latency=1}
      mask help:
      | An explicitly laid-out delay line to avoid mapping to SRL16s
      | for use in pipelining to help achieve timing closure.
      mask init:
      | pipeline_init(gcb, 'latency', latency);
      mask Display:
      | port_label('input', 1, 'd');
      | port_label('output', 1, 'q');
      | disp(['Z^-', num2str(latency)]);
  dbuf_ct_bram : Subsystem  mask{length=12, numSpecs=2, numXeng=3}
      mask prompts: length "Length of Spectrums (2^?) (FFT_real_2x vector length)"; numSpecs "Number of Spectrums (2^?) (pkt size in 16bit complex dual-pol words)"; numXeng "Number of Xengines total (2^?)"
      mask help: Sram transpose using double buffering method, maximum size is 256 spectrums by 2048 channels!!
  fft2x_tvg : Subsystem  mask{length=12}
      mask prompts: length "FFT_real_2x vector length (2^?)"
  one_ant_a_time : Subsystem
  sram_tvg : Subsystem
  Out1 : Outport
  tag scope: ant12_pol12_reorder=global, sync_reorder=global
  wires:
  fft2x_tvg/1(dout) -> Delay3/1(d)
  fft2x_tvg/2(sync_out) -> Delay2/1(d)
  sram_tvg/1(dout) -> one_ant_a_time/1(din)
  sram_tvg/2(sync_out) -> one_ant_a_time/2(sync)
  dbuf_ct_bram/1(out) -> Delay79/1(d)
  dbuf_ct_bram/2(sync_out) -> Delay1/1(d)
  [use_sram_tvg] -> sram_tvg/3(use_tvg)
  one_ant_a_time/1(dout) -> [ant12_pol12_reorder]
  one_ant_a_time/2(sync_out) -> [sync_reorder]
  [use_fft_tvg] -> fft2x_tvg/3(use_tvg)
  [eq_out] -> fft2x_tvg/2(din)
  [sync_rnd] -> fft2x_tvg/1(sync)
  In1/1 -> Out1/1
  Delay79/1(q) -> sram_tvg/1(din)
  Delay1/1(q) -> sram_tvg/2(sync)
  Delay3/1(q) -> dbuf_ct_bram/1(din)
  Delay2/1(q) -> dbuf_ct_bram/2(sync_in)

== system roachf_2048ch/WGNs ==
  Constant : Constant  Value=0
  Constant2 : Constant  Value=0
  Mux : Mux  Inputs=2
  noise0 : Subsystem
  noise1 : Subsystem
  noise2 : Subsystem
  noise3 : Subsystem
  Out1 : Outport
  tag scope: n00=global, n01=global, n10=global, n11=global, n20=global, n21=global, n30=global, n31=global
  wires:
  noise0/1(n1) -> [n00]
  noise0/2(n2) -> [n01]
  noise1/1(n1) -> [n10]
  noise1/2(n2) -> [n11]
  noise2/1(n1) -> [n20]
  noise2/2(n2) -> [n21]
  noise3/1(n1) -> [n30]
  noise3/2(n2) -> [n31]
  [seed0] -> noise0/1(seed)
  [seed3] -> noise3/1(seed)
  [seed2] -> noise2/1(seed)
  [seed1] -> noise1/1(seed)
  [seed_ld] -> noise0/2(ld)
  [seed_ld] -> noise3/2(ld)
  [seed_ld] -> noise2/2(ld)
  [seed_ld] -> noise1/2(ld)
  Mux/1 -> Out1/1
  Constant/1 -> Mux/1
  Constant2/1 -> Mux/2

== system roachf_2048ch/control ==
  ctl_regs : Subsystem
  delay : Subsystem  mask{addr_offset=8195}
      mask prompts: addr_offset "Address"
      mask init:
      | start_addr = (addr_offset);
      | fmtstr = sprintf('Addr %d\n0x%04X', start_addr, start_addr);
      | set_param(gcb, 'AttributesFormatString', fmtstr);
      settings: AttributesFormatString=|
      | Addr 8195
      | 0x2003
  eq_coefs : Subsystem
  insel : Subsystem  mask{addr_offset=8194}
      mask prompts: addr_offset "Address"
      mask init:
      | start_addr = (addr_offset);
      | fmtstr = sprintf('Addr %d\n0x%04X', start_addr, start_addr);
      | set_param(gcb, 'AttributesFormatString', fmtstr);
      settings: AttributesFormatString=|
      | Addr 8194
      | 0x2002
  seed : Subsystem  mask{addr_offset=8196}
      mask prompts: addr_offset "Address"
      mask init:
      | start_addr = (addr_offset);
      | fmtstr = sprintf('Addr %d\n0x%04X', start_addr, start_addr);
      | set_param(gcb, 'AttributesFormatString', fmtstr);
      settings: AttributesFormatString=|
      | Addr 8196
      | 0x2004

== system roachf_2048ch/input_mux ==
  In1 : Inport
  In2 : Inport  Port=2
  Delay : xbsIndex_r4/Delay  rst=off  infoeditControl=Selection of Reset will increase slice count due to use of real FFs and instead of SRLs  en=off  latency=2  dbl_ovrd=off  reg_retiming=off  block_type=delay
  Terminator : Terminator
  muxin0 : Subsystem
  muxin1 : Subsystem
  muxin2 : Subsystem
  muxin3 : Subsystem
  muxin4 : Subsystem
  muxin5 : Subsystem
  muxin6 : Subsystem
  muxin7 : Subsystem
  Out1 : Outport
  tag scope: in0=global, in1=global, in2=global, in3=global, in4=global, in5=global, in6=global, in7=global, mux_mon=global, pfb_sync=global
  wires:
  [insel0] -> muxin0/1(sel)
  [adc0] -> muxin0/2(adc)
  [n00] -> muxin0/3(n0), muxin1/3(n0)
  [n01] -> muxin0/4(n1), muxin1/4(n1)
  [delay0] -> muxin0/5(delay)
  muxin0/1(out) -> [in0], [mux_mon]
  [insel1] -> muxin1/1(sel)
  [adc1] -> muxin1/2(adc)
  [delay1] -> muxin1/5(delay)
  [insel2] -> muxin2/1(sel)
  [adc2] -> muxin2/2(adc)
  [n10] -> muxin3/3(n0), muxin2/3(n0)
  [n11] -> muxin3/4(n1), muxin2/4(n1)
  [delay2] -> muxin2/5(delay)
  [insel3] -> muxin3/1(sel)
  [adc3] -> muxin3/2(adc)
  [delay3] -> muxin3/5(delay)
  muxin1/1(out) -> [in1]
  muxin2/1(out) -> [in2]
  muxin3/1(out) -> [in3]
  [insel4] -> muxin4/1(sel)
  [adc4] -> muxin4/2(adc)
  [n20] -> muxin5/3(n0), muxin4/3(n0)
  [n21] -> muxin5/4(n1), muxin4/4(n1)
  [delay4] -> muxin4/5(delay)
  [insel5] -> muxin5/1(sel)
  [adc5] -> muxin5/2(adc)
  [delay5] -> muxin5/5(delay)
  [insel6] -> muxin6/1(sel)
  [adc6] -> muxin6/2(adc)
  [n30] -> muxin7/3(n0), muxin6/3(n0)
  [n31] -> muxin7/4(n1), muxin6/4(n1)
  [delay6] -> muxin6/5(delay)
  [insel7] -> muxin7/1(sel)
  [adc7] -> muxin7/2(adc)
  [delay7] -> muxin7/5(delay)
  muxin7/1(out) -> [in7]
  muxin4/1(out) -> [in4]
  muxin5/1(out) -> [in5]
  muxin6/1(out) -> [in6]
  [sync_gen] -> Delay/1
  Delay/1 -> [pfb_sync]
  In1/1 -> Out1/1
  In2/1 -> Terminator/1

== system roachf_2048ch/status ==
  Concat : xbsIndex_r4/Concat  num_inputs=8  dbl_ovrd=off  block_type=concat
  Concat1 : xbsIndex_r4/Concat  num_inputs=8  dbl_ovrd=off  block_type=concat
  Constant1 : xbsIndex_r4/Constant  const=0  gui_display_data_type=Fixed-point  arith_type=Unsigned  n_bits=25  bin_pt=0  preci_type=Single  exp_width=8  frac_width=24  explicit_period=on  period=1  equ=P=C  opselect=C  inp2=PCIN>>17  opr=+  inp1=P  carry=CIN  dbl_ovrd=off  block_type=constant
      settings: block_version=11.4
  Constant2 : xbsIndex_r4/Constant  const=0  gui_display_data_type=Fixed-point  arith_type=Unsigned  n_bits=25  bin_pt=0  preci_type=Single  exp_width=8  frac_width=24  explicit_period=on  period=1  equ=P=C  opselect=C  inp2=PCIN>>17  opr=+  inp1=P  carry=CIN  dbl_ovrd=off  block_type=constant
      settings: block_version=11.4
  gbe_gpu : xps_library/software register  Tag=xps:sw_reg  SystemSampleTime=-1  io_dir=To Processor  arith_type=Unsigned  bitwidth=32  bin_pt=0  sample_period=1  gw_name=roachf_2048ch_status_gbe_gpu_user_data_in
  gbe_sw : xps_library/software register  Tag=xps:sw_reg  SystemSampleTime=-1  io_dir=To Processor  arith_type=Unsigned  bitwidth=32  bin_pt=0  sample_period=1  gw_name=roachf_2048ch_status_gbe_sw_user_data_in
  wires:
  Concat/1 -> gbe_sw/1
  Constant1/1 -> Concat/1
  [gbe_sw_led_up] -> Concat/2
  [gbe_sw_led_rx] -> Concat/3
  [gbe_sw_led_tx] -> Concat/4
  [gbe_sw_tx_afull] -> Concat/5
  [gbe_sw_tx_oflow] -> Concat/6
  [gbe_sw_rx_bfr] -> Concat/7
  [gbe_sw_rx_orun] -> Concat/8
  Concat1/1 -> gbe_gpu/1
  Constant2/1 -> Concat1/1
  [gbe_gpu_led_up] -> Concat1/2
  [gbe_gpu_led_rx] -> Concat1/3
  [gbe_gpu_led_tx] -> Concat1/4
  [gbe_gpu_tx_ack] -> Concat1/5
  [gbe_gpu_rx_valid] -> Concat1/6
  [gbe_gpu_rx_eof] -> Concat1/7
  [gbe_gpu_rx_eof] -> Concat1/8
